simulink model "ukol_7_model"  (R2016a)
settings: Solver=VariableStepAuto  SolverMode=SingleTasking  StartTime=0.0  StopTime=10.0  RelTol=1e-3
libraries: cstblocks x2
settings Model: Creator=tomas  LastModifiedBy=tomas
settings DebuggingCC: SFUnexpectedBacktrackingDiag=error  SFNoUnconditionalDefaultTransitionDiag=error
settings GRTTargetCC: TargetLangStandard=C99 (ISO)  GeneratePreprocessorConditionals=Use local settings
settings ConfigComp: CovMetricSettings=dwe  CovHtmlReporting=off  CovSaveCumulativeToWorkspaceVar=off  CovSaveSingleToWorkspaceVar=off  CovExternalEMLEnable=on

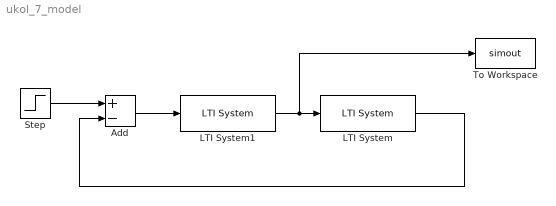
== system ukol_7_model ==
  Add : Sum  Inputs=+-
  LTI System : cstblocks/LTI System  sys=Fs_servo_discrete  IC=[]
  LTI System1 : cstblocks/LTI System  sys=Fr_7  IC=[]
  Step : Step  SampleTime=0
  To Workspace : ToWorkspace  VariableName=simout  SaveFormat=Timeseries  SampleTime=-1
  wires:
  LTI System1/1 -> To Workspace/1, LTI System/1
  Add/1 -> LTI System1/1
  LTI System/1 -> Add/2
  Step/1 -> Add/1
